simulink model "x1sim"  (Simulink 9.3)
settings: Solver=ode45  StartTime=0.0  StopTime=10.0  RelTol=1e-3  EnableMultiTasking=on
libraries: cdsFilt x6, cdsGaussianNoiseGenerator x2, cdsAdcx0 x1, cdsEpicsMomentary x1, cdsParameters x1
settings Model: Creator=jkissel  LastModifiedBy=ccw
settings DataIOCC: LimitDataPoints=on
settings OptimizationCC: ExpressionDepthLimit=2147483647
settings DebuggingCC: SolverPrmCheckMsg=warning  AllowSymbolicDim=off  StateNameClashWarn=warning

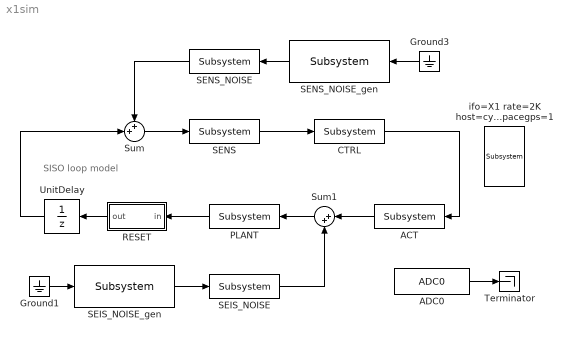
== system x1sim ==
  note: SISO loop model
  ACT : cdsFilt/Subsystem  Tag=cdsFilt  Description=|  SystemSampleTime=-1  Latency=0  AutoFrameSizeCalculation=off
      | Purpose:                                                                                                                                                                                                                                  
      | Standard CDS IIR filter module.                                                                                                                                                                                                           
      |                                                                                                                                                                                                                                           
      | Operation:                                                                                                                                                                                                                                
      | Consists of 10 second order section IIR filters, plus a ramped gain stage. In FE code, also provides pre-defined test points and excitation channel inputs. The filter coefficients are defined in the LIGO system using the 'foton' tool.
      |                                                                                                                                                                                                                                           
      | Usage:                                                                                                                                                                                                                                    
      | Name the part with the desired filter module name.
      settings: AttributesFormatString=%<Tag>
  ADC0 : cdsAdcx0/ADC0  Tag=cdsAdc  Description=|  SystemSampleTime=-1  Latency=0  AutoFrameSizeCalculation=off
      | type-GSC_16AI64SSA
      | card_num=0
      settings: AttributesFormatString=%<Description>\n%<Tag>
  CTRL : cdsFilt/Subsystem  Tag=cdsFilt  Description=|  SystemSampleTime=-1  Latency=0  AutoFrameSizeCalculation=off
      | Purpose:                                                                                                                                                                                                                                  
      | Standard CDS IIR filter module.                                                                                                                                                                                                           
      |                                                                                                                                                                                                                                           
      | Operation:                                                                                                                                                                                                                                
      | Consists of 10 second order section IIR filters, plus a ramped gain stage. In FE code, also provides pre-defined test points and excitation channel inputs. The filter coefficients are defined in the LIGO system using the 'foton' tool.
      |                                                                                                                                                                                                                                           
      | Usage:                                                                                                                                                                                                                                    
      | Name the part with the desired filter module name.
      settings: AttributesFormatString=%<Tag>
  Ground1 : Ground
  Ground3 : Ground
  PLANT : cdsFilt/Subsystem  Tag=cdsFilt  Description=|  SystemSampleTime=-1  Latency=0  AutoFrameSizeCalculation=off
      | Purpose:                                                                                                                                                                                                                                  
      | Standard CDS IIR filter module.                                                                                                                                                                                                           
      |                                                                                                                                                                                                                                           
      | Operation:                                                                                                                                                                                                                                
      | Consists of 10 second order section IIR filters, plus a ramped gain stage. In FE code, also provides pre-defined test points and excitation channel inputs. The filter coefficients are defined in the LIGO system using the 'foton' tool.
      |                                                                                                                                                                                                                                           
      | Usage:                                                                                                                                                                                                                                    
      | Name the part with the desired filter module name.
      settings: AttributesFormatString=%<Tag>
  RESET : Subsystem
  SEIS_NOISE : cdsFilt/Subsystem  Tag=cdsFilt  Description=|  SystemSampleTime=-1  Latency=0  AutoFrameSizeCalculation=off
      | Purpose:                                                                                                                                                                                                                                  
      | Standard CDS IIR filter module.                                                                                                                                                                                                           
      |                                                                                                                                                                                                                                           
      | Operation:                                                                                                                                                                                                                                
      | Consists of 10 second order section IIR filters, plus a ramped gain stage. In FE code, also provides pre-defined test points and excitation channel inputs. The filter coefficients are defined in the LIGO system using the 'foton' tool.
      |                                                                                                                                                                                                                                           
      | Usage:                                                                                                                                                                                                                                    
      | Name the part with the desired filter module name.
      settings: AttributesFormatString=%<Tag>
  SEIS_NOISE_gen : cdsGaussianNoiseGenerator/Subsystem  Tag=cdsGaussianNoiseGenerator  SystemSampleTime=-1  Latency=0  AutoFrameSizeCalculation=off
      settings: AttributesFormatString=%<Tag>
  SENS : cdsFilt/Subsystem  Tag=cdsFilt  Description=|  SystemSampleTime=-1  Latency=0  AutoFrameSizeCalculation=off
      | Purpose:                                                                                                                                                                                                                                  
      | Standard CDS IIR filter module.                                                                                                                                                                                                           
      |                                                                                                                                                                                                                                           
      | Operation:                                                                                                                                                                                                                                
      | Consists of 10 second order section IIR filters, plus a ramped gain stage. In FE code, also provides pre-defined test points and excitation channel inputs. The filter coefficients are defined in the LIGO system using the 'foton' tool.
      |                                                                                                                                                                                                                                           
      | Usage:                                                                                                                                                                                                                                    
      | Name the part with the desired filter module name.
      settings: AttributesFormatString=%<Tag>
  SENS_NOISE : cdsFilt/Subsystem  Tag=cdsFilt  Description=|  SystemSampleTime=-1  Latency=0  AutoFrameSizeCalculation=off
      | Purpose:                                                                                                                                                                                                                                  
      | Standard CDS IIR filter module.                                                                                                                                                                                                           
      |                                                                                                                                                                                                                                           
      | Operation:                                                                                                                                                                                                                                
      | Consists of 10 second order section IIR filters, plus a ramped gain stage. In FE code, also provides pre-defined test points and excitation channel inputs. The filter coefficients are defined in the LIGO system using the 'foton' tool.
      |                                                                                                                                                                                                                                           
      | Usage:                                                                                                                                                                                                                                    
      | Name the part with the desired filter module name.
      settings: AttributesFormatString=%<Tag>
  SENS_NOISE_gen : cdsGaussianNoiseGenerator/Subsystem  Tag=cdsGaussianNoiseGenerator  SystemSampleTime=-1  Latency=0  AutoFrameSizeCalculation=off
      settings: AttributesFormatString=%<Tag>
  Sum : Sum  Inputs=++|
  Sum1 : Sum  Inputs=|++
  Terminator : Terminator
  UnitDelay : UnitDelay  SampleTime=-1  HasFrameUpgradeWarning=on
  ifo=X1 rate=2K host=cymac dcuid=8 specific_cpu=3 userspacegps=1 : cdsParameters/Subsystem  Tag=cdsParameters  Description=|  SystemSampleTime=-1  Latency=0  AutoFrameSizeCalculation=off
      | Purpose:                                                                                                                                                                                                                                
      | Provide system parameters to the FE code generator to properly configure the generated EPICS names, rep rate of the FE controller, and the Data Acquisition node ID for proper storage of data from this FE controller.                 
      |                                                                                                                                                                                                                                         
      | Useage:                                                                                                                                                                                                                                 
      | The part NAME field is used to identify the FE parameters. It must be of the form:                                                                                                                                                      
      | site=                                                                                                                                                                                                                                   
      | rate=                                                                                                                                                                                                                                   
      | dcuid=                                                                                                                                                                                                                                  
      |                                                                                                                                                                                                                                         
      | Where:                                                                                                                                                                                                                                  
      | site= argument may be H1, H2, L1, M1, G1, either as a single argument or multiple, for example site=H1,H2. These are the only names allowed. These will become the first two characters of all EPICS and signal names (for example G1:).
      |                                                                                                                                                                                                                                         
      | rate= may be 2K, 16K, 32K, or 64K                                                                                                                                                                                                       
      |                                                                                                                                                                                                                                         
      | dcuid= is site specific ie it must be unique at each site.
      settings: AttributesFormatString=%<Tag>
  wires:
  ADC0/1 -> Terminator/1
  RESET/1(out) -> UnitDelay/1
  SENS_NOISE_gen/1 -> SENS_NOISE/1
  SENS/1 -> CTRL/1
  Sum/1 -> SENS/1
  SENS_NOISE/1 -> Sum/1
  CTRL/1 -> ACT/1
  PLANT/1 -> RESET/1(in)
  SEIS_NOISE_gen/1 -> SEIS_NOISE/1
  Ground1/1 -> SEIS_NOISE_gen/1
  Sum1/1 -> PLANT/1
  ACT/1 -> Sum1/1
  SEIS_NOISE/1 -> Sum1/2
  UnitDelay/1 -> Sum/2
  Ground3/1 -> SENS_NOISE_gen/1

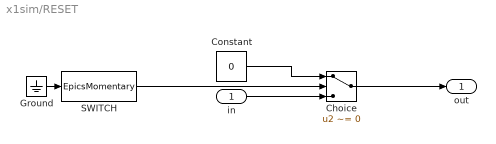
== system x1sim/RESET ==
  in : Inport
  Choice : Switch  Criteria=u2 ~= 0
  Constant : Constant  Value=0
  Ground : Ground
  SWITCH : cdsEpicsMomentary/EpicsMomentary  Tag=cdsEpicsMomentary  SystemSampleTime=-1  Latency=0  AutoFrameSizeCalculation=off
      settings: AttributesFormatString=%<Tag>
  out : Outport
  wires:
  in/1 -> Choice/3
  Choice/1 -> out/1
  Constant/1 -> Choice/1
  SWITCH/1 -> Choice/2
  Ground/1 -> SWITCH/1
